simulink model "sl_groundvehicleDynamics"  (R2024a)
settings: Solver=ode45  StartTime=0.0  StopTime=5000  RelTol=1e-5  EnableMultiTasking=on
InitFcn:
  | [waypoints,waypoint_mat,path] = wpMap;
undefined symbols (not defined in the file or in its folder): waypoint_mat, waypoints
libraries: simulink x4, mobileRoboticsLib x3, simulink_extras x2
settings Model: PacingRate=10  Creator=sriramn  LastModifiedBy=Cam
settings SolverCC: ZeroCrossAlgorithm=Adaptive  AlgebraicLoopSolver=TrustRegion
settings DataIOCC: LimitDataPoints=on  SaveFormat=Array  ReturnWorkspaceOutputs=off
settings OptimizationCC: ReuseModelBlockBuffer=off  LifeSpan=inf
settings DebuggingCC: AlgebraicLoopMsg=none  SolverPrmCheckMsg=warning  UnconnectedInputMsg=warning  UnconnectedOutputMsg=warning  UnconnectedLineMsg=warning  AllowSymbolicDim=off  SFUnexpectedBacktrackingDiag=warning  SFNoUnconditionalDefaultTransitionDiag=warning  SFExecutionAtInitializationDiag=none  ArithmeticOperatorsInVariantConditions=warning
settings ModelReferenceCC: EnableRefExpFcnMdlSchedulingChecks=on  ModelReferenceMinAlgLoopOccurrences=on  PropagateSignalLabelsOutOfModel=off
settings SFSimCC: SimUseLocalCustomCode=off  CustomCodeUndefinedFunction=UseInterfaceOnly
settings RTWCC: RTWUseLocalCustomCode=off  GPUComputeCapability=3.5
settings CodeAppCC: StateflowObjectComments=on
settings GRTTargetCC: TargetLangStandard=C89/C90 (ANSI)
settings ConfigComp: CovMetricSettings=dw  CovSaveCumulativeToWorkspaceVar=on  CovSaveSingleToWorkspaceVar=on  CovExternalEMLEnable=off  CovSFcnEnable=off
settings SimscapeCC: SimscapeNormalizeSystem=off
settings ConfigurationSet: Description=SimMechanics 2G
settings ExplorerConfigSet: InternalSimMechanicsExplorerSettings="<ExplorerConfiguration><canonicalview>planar_xy</canonicalview><AnimationSetting><BasePlaybackSpeed>1.0</BasePlaybackSpeed><PlaybackSpeedFactor>1.0</PlaybackSpeedFactor></AnimationSetting><TilePanel><TileInfo><Tiles Columns=\"1\" Count=\"1\" Rows=\"1\"><Column Left=\"2\" Weight=\"1\"/><Column Left=\"1628\"/><Row Top=\"2\" Weight=\"1\"/><Row Top=\"1072\"/><Tile Height=\"1\" Width=\"1\" X=\"0\" Y=\"0\"/></Tiles></TileInfo><SceneInfo><SceneViewer><BGColor><R>0.60000002384185791</R><G>0.60000002384185791</G><B>0.60000002384185791</B></BGColor><Camera><Position><X>0.22951840878551699</X><Y>0.32651610611526627</Y><Z>-0.27215421354393321</Z></Position><Center><X>-0.15775714411666431</X><Y>-0.15462825985839526</Y><Z>0.065702552916005602</Z></Center><Up><X>-0.56030137557930915</X><Y>0.72817587161684794</Y><Z>0.39474329445726858</Z></Up><Left>-0.21481383955700509</Left><Right>0.21481383955700509</Right><Bottom>-0.27569784609469139</Bottom><Top>0.27569784609469139</Top></Camera></SceneViewer></SceneInfo></TilePanel></ExplorerConfiguration>"

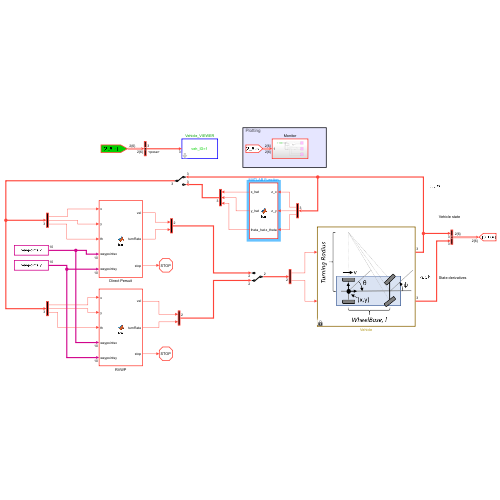
[thumbnail: Simulink's stored preview of the top-level diagram]
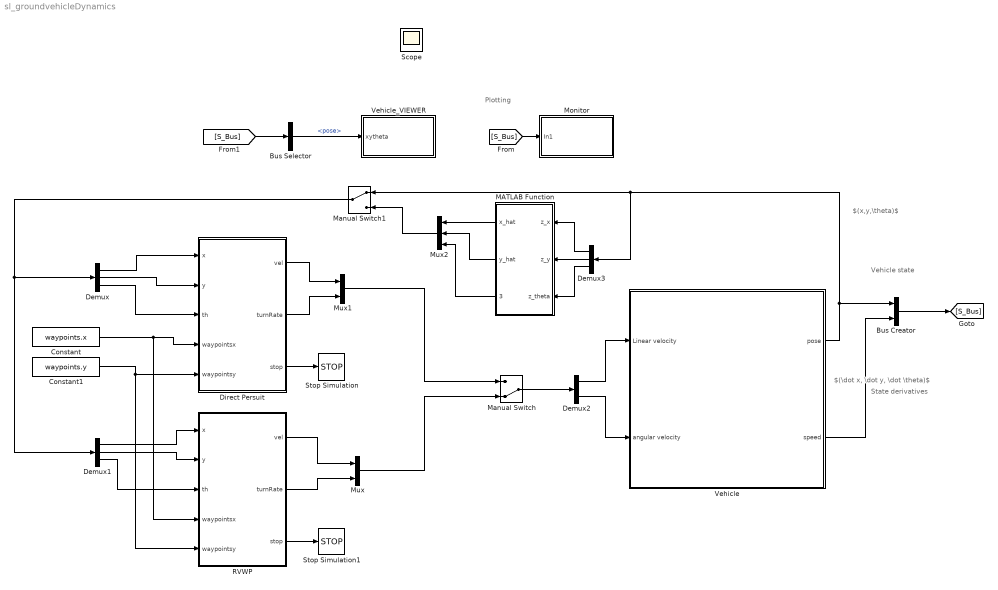
== system sl_groundvehicleDynamics ==
  note: State derivatives
  note: $(x,y,\theta)$
  note: $(\dot x, \dot y, \dot \theta)$
  note: Vehicle state
  note: Plotting
  Bus Creator : BusCreator  Inputs=2
  Bus Selector : BusSelector  OutputSignals=pose
  Constant : Constant  Value=waypoints.x
  Constant1 : Constant  Value=waypoints.y
  Demux : Demux  Outputs=3
  Demux1 : Demux  Outputs=3
  Demux2 : Demux  Outputs=2
  Demux3 : Demux  Outputs=3
  Direct Persuit : MATLAB Function  TreatAsAtomicUnit=on
  MATLAB Function : MATLAB Function  TreatAsAtomicUnit=on
  Manual Switch : ManualSwitch  CurrentSetting=0
  Manual Switch1 : ManualSwitch
  Monitor : Subsystem
  Mux : Mux  Inputs=2
  Mux1 : Mux  Inputs=2
  Mux2 : Mux  Inputs=3
  RVWP : MATLAB Function  TreatAsAtomicUnit=on
  Stop Simulation : Stop
  Stop Simulation1 : Stop
  Vehicle : Subsystem
      mask Display: image('$imagefile'); % Use "Edit Image" on toolstrip to change.
  Vehicle_VIEWER : Subsystem  mask{wp_mat=waypoint_mat, veh_ID_num=1, veh_init_xytheta=[0,0,0], Ts=0.5}
      mask prompts: wp_mat "Waypoint matrix for arena [x_col, y_col] (m)"; veh_ID_num "Vehicle ID number"; veh_init_xytheta "Initial pose [x,y,theta]"; Ts "Sample time for updating animation (secs)"
      mask TypeOptions veh_ID_num: 1 | 2 | 3 | 4
      mask DialogControl Control2 Prompt: Animate simulation of Differential Drive Robot (DDR)
      mask Display: fprintf('veh_ID=%d',veh_ID_num);
  Scope : Scope
  wires:
  [S_Bus] -> Monitor/1(In1)
  [S_Bus] -> Bus Selector/1
  Direct Persuit/1(vel) -> Mux1/1
  Vehicle/1(pose) -> Demux3/1, Manual Switch1/1, Bus Creator/1
  Vehicle/2(speed) -> Bus Creator/2
  Bus Creator/1 -> [S_Bus]
  Bus Selector/1 -> Vehicle_VIEWER/1(xytheta)  "<pose>"
  Direct Persuit/2(turnRate) -> Mux1/2
  Constant/1 -> RVWP/4(waypointsx), Direct Persuit/4(waypointsx)
  Demux/3 -> Direct Persuit/3(th)
  Demux/2 -> Direct Persuit/2(y)
  Demux/1 -> Direct Persuit/1(x)
  Constant1/1 -> RVWP/5(waypointsy), Direct Persuit/5(waypointsy)
  Direct Persuit/3(stop) -> Stop Simulation/1
  Demux1/1 -> RVWP/1(x)
  Demux1/2 -> RVWP/2(y)
  Demux1/3 -> RVWP/3(th)
  RVWP/3(stop) -> Stop Simulation1/1
  RVWP/1(vel) -> Mux/1
  RVWP/2(turnRate) -> Mux/2
  Mux/1 -> Manual Switch/2
  Mux1/1 -> Manual Switch/1
  Manual Switch/1 -> Demux2/1
  Demux2/1 -> Vehicle/1(Linear velocity)
  Demux2/2 -> Vehicle/2(angular velocity)
  Demux3/1 -> MATLAB Function/1(z_x)
  Demux3/2 -> MATLAB Function/2(z_y)
  Demux3/3 -> MATLAB Function/3(z_theta)
  Mux2/1 -> Manual Switch1/2
  Manual Switch1/1 -> Demux1/1, Demux/1
  MATLAB Function/1(x_hat) -> Mux2/1
  MATLAB Function/2(y_hat) -> Mux2/2
  MATLAB Function/3(theta_hat) -> Mux2/3

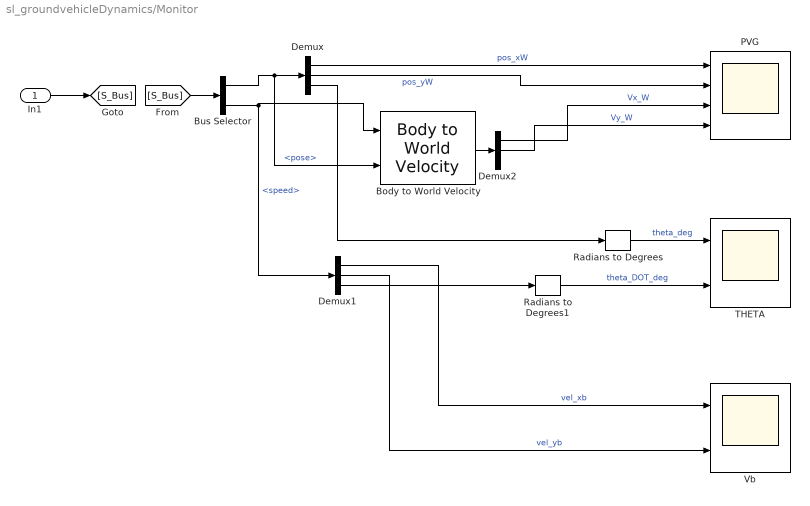
== system sl_groundvehicleDynamics/Monitor ==
  In1 : Inport
  Body to World Velocity : mobileRoboticsLib/Utilities/Body to World Velocity
      settings: SourceProductName=Mobile Robotics Simulation Toolbox
  Bus Selector : BusSelector  OutputSignals=pose,speed
  Demux : Demux  Outputs=3
  Demux1 : Demux  Outputs=3
  Demux2 : Demux  Outputs=3
  PVG : Scope  NumInputPorts=4
  Radians to Degrees : simulink_extras/Transformations/Radians to Degrees
  Radians to Degrees1 : simulink_extras/Transformations/Radians to Degrees
  THETA : Scope  NumInputPorts=2
  Vb : Scope  NumInputPorts=2
  wires:
  In1/1 -> [S_Bus]
  [S_Bus] -> Bus Selector/1
  Demux/1 -> PVG/1  "pos_xW"
  Demux/2 -> PVG/2  "pos_yW"
  Radians to Degrees1/1 -> THETA/2  "theta_DOT_deg"
  Radians to Degrees/1 -> THETA/1  "theta_deg"
  Demux1/3 -> Radians to Degrees1/1
  Demux/3 -> Radians to Degrees/1
  Bus Selector/1 -> Body to World Velocity/2, Demux/1  "<pose>"
  Bus Selector/2 -> Demux1/1, Body to World Velocity/1  "<speed>"
  Body to World Velocity/1 -> Demux2/1
  Demux2/1 -> PVG/3  "Vx_W"
  Demux2/2 -> PVG/4  "Vy_W"
  Demux1/1 -> Vb/1  "vel_xb"
  Demux1/2 -> Vb/2  "vel_yb"

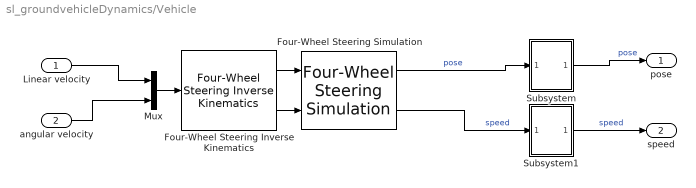
== system sl_groundvehicleDynamics/Vehicle ==
  Linear velocity : Inport
  angular velocity : Inport  Port=2
  Four-Wheel Steering Inverse Kinematics : mobileRoboticsLib/Kinematic Models/Four-Wheel Steering/Four-Wheel Steering Inverse Kinematics  wheelRadius=0.1  frontWheelDist=0.25  rearWheelDist=0.25  ikMode=Front Steering
      settings: SourceProductName=Mobile Robotics Simulation Toolbox
  Four-Wheel Steering Simulation : mobileRoboticsLib/Kinematic Models/Four-Wheel Steering/Four-Wheel Steering Simulation  wheelRadius=0.1  frontWheelDist=0.25  rearWheelDist=0.25  initX=0  initY=0  initAngle=0  Ts=0.05
      settings: SourceProductName=Mobile Robotics Simulation Toolbox
  Mux : Mux  Inputs=2
  Subsystem : Subsystem
  Subsystem1 : Subsystem
  pose : Outport  VectorParamsAs1DForOutWhenUnconnected=off
  speed : Outport  Port=2
  wires:
  angular velocity/1 -> Mux/2
  Linear velocity/1 -> Mux/1
  Mux/1 -> Four-Wheel Steering Inverse Kinematics/1
  Four-Wheel Steering Simulation/1 -> Subsystem/1(In1)  "pose"
  Four-Wheel Steering Simulation/2 -> Subsystem1/1(In1)  "speed"
  Four-Wheel Steering Inverse Kinematics/1 -> Four-Wheel Steering Simulation/1
  Four-Wheel Steering Inverse Kinematics/2 -> Four-Wheel Steering Simulation/2
  Subsystem/1(pose) -> pose/1  "pose"
  Subsystem1/1(speed) -> speed/1  "speed"

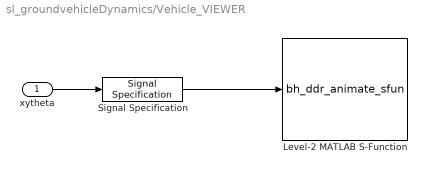
== system sl_groundvehicleDynamics/Vehicle_VIEWER ==
  xytheta : Inport
  Level-2 MATLAB S-Function : M-S-Function  FunctionName=bh_ddr_animate_sfun  Parameters=Ts, wp_mat, veh_ID_num, veh_init_xytheta
  Signal Specification : SignalSpecification  Dimensions=3
  wires:
  xytheta/1 -> Signal Specification/1
  Signal Specification/1 -> Level-2 MATLAB S-Function/1

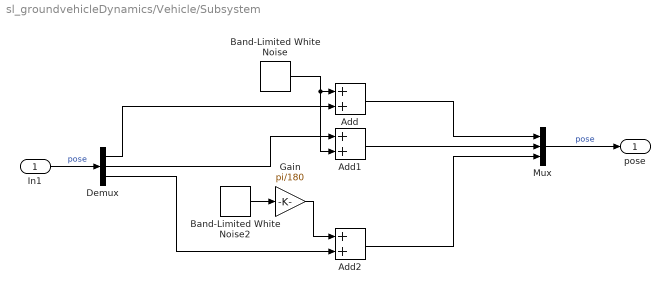
== system sl_groundvehicleDynamics/Vehicle/Subsystem ==
  In1 : Inport
  Add : Sum
  Add1 : Sum
  Add2 : Sum
  Band-Limited White Noise : simulink/Sources/Band-Limited White Noise  Cov=[0.001]  Ts=0.1  seed=[23341]
  Band-Limited White Noise2 : simulink/Sources/Band-Limited White Noise  Cov=[0.41]  Ts=0.1  seed=[23341]
  Demux : Demux  Outputs=3
  Gain : Gain  Gain=pi/180
  Mux : Mux  Inputs=3
  pose : Outport
  wires:
  Add1/1 -> Mux/2
  Add2/1 -> Mux/3
  Demux/2 -> Add1/1
  Band-Limited White Noise2/1 -> Gain/1
  Demux/3 -> Add2/2
  Band-Limited White Noise/1 -> Add1/2, Add/1
  In1/1 -> Demux/1  "pose"
  Demux/1 -> Add/2
  Gain/1 -> Add2/1
  Mux/1 -> pose/1  "pose"
  Add/1 -> Mux/1

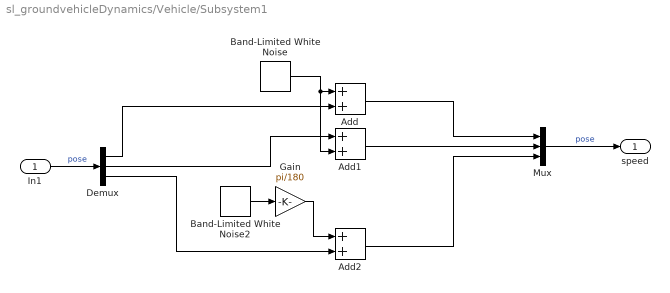
== system sl_groundvehicleDynamics/Vehicle/Subsystem1 ==
  In1 : Inport
  Add : Sum
  Add1 : Sum
  Add2 : Sum
  Band-Limited White Noise : simulink/Sources/Band-Limited White Noise  Cov=[0.001]  Ts=0.1  seed=[23341]
  Band-Limited White Noise2 : simulink/Sources/Band-Limited White Noise  Cov=[0.41]  Ts=0.1  seed=[23341]
  Demux : Demux  Outputs=3
  Gain : Gain  Gain=pi/180
  Mux : Mux  Inputs=3
  speed : Outport
  wires:
  Add1/1 -> Mux/2
  Add2/1 -> Mux/3
  Demux/2 -> Add1/1
  Band-Limited White Noise2/1 -> Gain/1
  Demux/3 -> Add2/2
  Band-Limited White Noise/1 -> Add1/2, Add/1
  In1/1 -> Demux/1  "pose"
  Demux/1 -> Add/2
  Gain/1 -> Add2/1
  Mux/1 -> speed/1  "pose"
  Add/1 -> Mux/1

== matlab function sl_groundvehicleDynamics/RVWP ==
  data: x input; y input; th input; waypointsx input; waypointsy input; vel output; turnRate output; stop output
function [vel,turnRate,stop] = fcn(x,y,th,waypointsx,waypointsy)


persistent WpCounter;
if isempty(WpCounter)
    WpCounter = 1; %% next waypoint
end

persistent Wpprev;
if isempty(Wpprev)
    Wpprev = WpCounter-1; %% waypoint ur currently at
end

 
if(Wpprev == 0)
    Next_wp = [waypointsx(WpCounter),waypointsy(WpCounter)];
    Prev_wp = [0,0];
 else
     Next_wp = [waypointsx(WpCounter),waypointsy(WpCounter)];
     Prev_wp = [waypointsx(Wpprev),waypointsy(Wpprev)];
     %Prev_wp = [0,0];
 end

dist2target = sqrt((Next_wp(2)-y)^2+(Next_wp(1)-x)^2);
distwp2wp = sqrt((Next_wp(2)-Prev_wp(2))^2+(Next_wp(1)-Prev_wp(1))^2);
dist2Last = sqrt((Prev_wp(2)-y)^2+(Prev_wp(1)-x)^2);
unitvec = [Next_wp(1)-Prev_wp(1),Next_wp(2)-Prev_wp(2)]/distwp2wp;

sigma = 10;
targetrel = (dist2Last+10)*unitvec;
target = [targetrel(1)+Prev_wp(1),targetrel(2)+Prev_wp(2)];
thtarget = atan2(target(2)-y,target(1)-x);


%% --- Control Shit ------ 
error = angdiff(th,thtarget);
K_theta = 0.5;
omega = K_theta * error;  % proportional control  - omega is the command
turnRate = omega;


persistent velocity;
if isempty(velocity)
    velocity = 0.5;
end
if(dist2target > 25)
    velocity = velocity+0.001;
    if(velocity >1)
        velocity = 1;
    end
else
    velocity = velocity-0.001;
    if(velocity < 3)
        velocity = 3; 
    end
end
vel = 3;

if(dist2target <= 2)
    Wpprev = WpCounter;
    WpCounter = WpCounter+1;

    if(WpCounter > 10)
        stop = 1;
    else 
        stop = 0;
    end
else    
    stop = 0;
end

== matlab function sl_groundvehicleDynamics/Direct Persuit ==
  data: x input; y input; th input; waypointsx input; waypointsy input; vel output; turnRate output; stop output
function [vel,turnRate,stop] = fcn(x,y,th,waypointsx,waypointsy)

persistent WpCounter;
if isempty(WpCounter)
    WpCounter = 1;
end

dist2Target = sqrt((waypointsx(WpCounter)-x)^2 + (waypointsy(WpCounter)-y)^2); %%Ru
location_current = [x,y];

location_star = [waypointsx(WpCounter),waypointsy(WpCounter)];
delta_location = location_star-location_current;
theta_star = atan2(delta_location(2),delta_location(1));  % Required heading to the waypoint

error = angdiff(th,theta_star);
K_theta = 0.05;
omega = K_theta * error;  % proportional control  - omega is the command
turnRate = omega;

persistent velocity;
if isempty(velocity)
    velocity = 0.5;
end
if(dist2Target > 25)
    velocity = velocity+0.001;
    if(velocity >1)
        velocity = 1;
    end
else
    velocity = velocity-0.001;
    if(velocity <0.5)
        velocity = 0.5; 
    end
end
vel = velocity;

if(dist2Target <= 10)
    WpCounter = WpCounter+1;
    if(WpCounter > 10)
        stop = 1;
    else 
        stop = 0;
    end
else    
    stop = 0;
end

== matlab function sl_groundvehicleDynamics/MATLAB Function ==
  data: z_x input; x_hat output; z_y input; z_theta input; y_hat output; theta_hat output
function [x_hat, y_hat, theta_hat] = fcn(z_x, z_y, z_theta)
    %% define time step for filter     
    persistent ts;
    if isempty(ts)
        ts = 0;
    end

    persistent prev_ts;
    if isempty(prev_ts)
        prev_ts = 0;
    end

    persistent step;
    if isempty(step)
        step = 0;
    end

    if (step > 0)
        prev_ts = ts - 0.1;
    end

    % Pre-allocate a bunch of persistent shit...
    persistent z_ts;
    if isempty(z_ts)
        % Pre-allocate a large array of z for sampling
        z_ts = zeros(3, 1000000);
    end

    persistent R_1;
    if (isempty(R_1))
        R_1 = zeros(3, 3);
    end

    persistent x_1;
    if (isempty(x_1))
        x_1 = zeros(6, 1);
    end

    persistent P_1;
    if (isempty(P_1))
        P_1 = zeros(6, 6);
    end

    persistent R_2;
    if (isempty(R_2))
        R_2 = zeros(6, 6);
    end

    persistent x_2;
    if (isempty(x_2))
        x_2 = zeros(6, 1);
    end

    persistent P_2;
    if (isempty(P_2))
        P_2 = zeros(6, 6);
    end

    %% Initilize the System State Equations
    % Measurement Covariance Matrix
    sigma_x_measured = 0.1; % meteres
    sigma_y_measured = 0.1; % meteres
    sigma_theta_measured = 2; % degrees
    
    if step == 0
        % Set the measured values...
        z_ts(:, step + 1) = [ ...
             z_x; ...
             z_y; ...
             z_theta ...
        ];
    
        % Assume that there is no correlation between x, y & theta...
        R_1 = [sigma_x_measured, 0, 0; ...
               0, sigma_y_measured, 0; ...
               0, 0, sigma_theta_measured];

        x_1 = [z_x; ...
               z_y; ...
               z_theta; ...,
               0; ...
               0; ...
               0];
        
        P_1(1:3, 1:3) = R_1;
    end

    %% Re-Initilize the System State Equations
    if step == 1
        % Set the measured values...
        z_ts(:, step + 1) = [ ...
             z_x; ...
             z_y; ...
             z_theta ...
        ];
    
        % Assume that there is no correlation between x, y & theta...
        R_2 = [sigma_x_measured, 0, 0; ...
               0, sigma_y_measured, 0; ...
               0, 0, sigma_theta_measured];

        delta_t = ts - prev_ts;
        prev_state = z_ts(:, step + 1);

        x_2 = [z_x; ...
               z_y; ...
               z_theta; ...,
               (z_x - prev_state(1)) / delta_t; ...
               (z_y - prev_state(2)) / delta_t; ...
               (z_theta - prev_state(3)) / delta_t];
        
        P_2(1:3, 1:3) = R_2;
        P_2(4,4) = 1e5;
        P_2(5,5) = 1e5;
        P_2(6,6) = 1e5;
    end

    
    if step > 1

        delta_t = ts - prev_ts;
        
        A = [1, 0, 0, delta_t, 0, 0; ...
             0, 1, 0, 0, delta_t, 0; ...
             0, 0, 1, 0, 0, delta_t; ...
             0, 0, 0, 1, 0, 0; ...
             0, 0, 0, 0, 1, 0; ...
             0, 0, 0, 0, 0, 1; ...
            ];

        x_pred = A * x_2;
        P_pred = A * P_2 * A.';

        foo = [1; 1; 1];
        bar = [delta_t^2/2, delta_t^2/2, delta_t^2/2, delta_t, delta_t, delta_t];

        H = foo * bar;

        kalman_gain = (P_pred * H.') * (H * P_pred * H.' + R_2)^(-1);

        x_n = x_pred + kalman_gain * ([z_x; z_y; z_theta] - H * x_pred);
        P_n = P_pred - (kalman_gain * H * P_pred);

        %% return the estimated values
        x_hat = x_n(1);
        y_hat = x_n(2);
        theta_hat = x_n(3);

        % TODO - Fix the gain & P matrix estimation 
        P_2 = P_n;
        x_2 = x_n;
    
        % increment the time step...
        step = step + 1;
        ts = ts + 0.1;

        return
    end
    % Dont do anything for now...
    x_hat = z_x;
    y_hat = z_y;
    theta_hat = z_theta;

    % increment the time step...
    step = step + 1;
    ts = ts + 0.1;
end
